simulink model "Block_diagram"  (R2013a)
settings: Solver=ode45  StartTime=0.0  StopTime=10.0  RelTol=1e-3
settings Model: Creator=Raman  LastModifiedBy=Raman

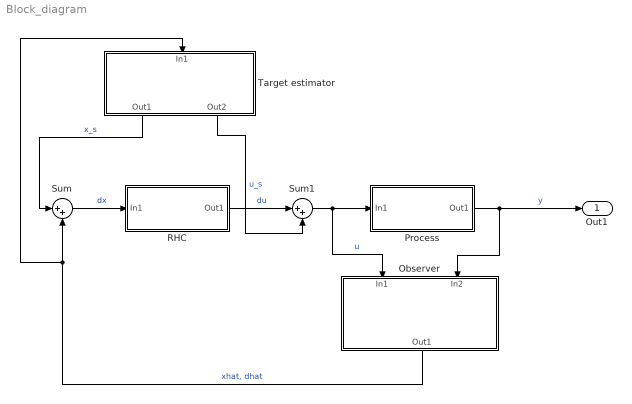
== system Block_diagram ==
  Observer : Subsystem
  Process : Subsystem
  RHC : Subsystem
  Sum : Sum  Inputs=|++
  Sum1 : Sum  Inputs=|++
  Target estimator : Subsystem
  Out1 : Outport
  wires:
  Sum/1 -> RHC/1(In1)  "dx"
  Target estimator/1(Out1) -> Sum/1  "x_s"
  Target estimator/2(Out2) -> Sum1/2  "u_s"
  RHC/1(Out1) -> Sum1/1  "du"
  Sum1/1 -> Process/1(In1), Observer/1(In1)  "u"
  Process/1(Out1) -> Observer/2(In2), Out1/1  "y"
  Observer/1(Out1) -> Target estimator/1(In1), Sum/2  "xhat, dhat"

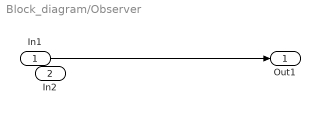
== system Block_diagram/Observer ==
  In1 : Inport
  In2 : Inport  Port=2
  Out1 : Outport
  wires:
  In1/1 -> Out1/1

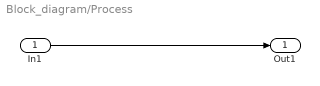
== system Block_diagram/Process ==
  In1 : Inport
  Out1 : Outport
  wires:
  In1/1 -> Out1/1

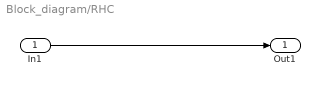
== system Block_diagram/RHC ==
  In1 : Inport
  Out1 : Outport
  wires:
  In1/1 -> Out1/1

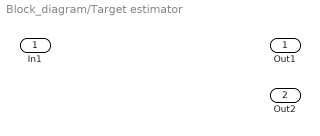
== system Block_diagram/Target estimator ==
  In1 : Inport
  Out1 : Outport
  Out2 : Outport  Port=2
